simulink model "test"  (R2017a)
settings: Solver=FixedStepAuto  StartTime=0.0  StopTime=Inf  FixedStep=5e-4  RelTol=1e-3  EnableMultiTasking=on
libraries: simulink x1
settings Model: SimulationMode=external  ExtModeTrigDuration=1000000  Creator=bbb  LastModifiedBy=Nils
settings DataIOCC: LimitDataPoints=on  SaveFormat=Array
settings OptimizationCC: PassReuseOutputArgsAs=Individual arguments
settings DebuggingCC: SolverPrmCheckMsg=warning  ParameterTunabilityLossMsg=error  SFUnexpectedBacktrackingDiag=warning  SFNoUnconditionalDefaultTransitionDiag=warning  SFExecutionAtInitializationDiag=none
settings HardwareCC: ProdBitPerPointer=32  ProdBitPerSizeT=32  ProdBitPerPtrDiffT=32  ProdLargestAtomicFloat=None  ProdIntDivRoundTo=Undefined  ProdEndianess=Unspecified  ProdWordSize=32  ProdHWDeviceType=32-bit Generic
settings ModelReferenceCC: PropagateSignalLabelsOutOfModel=off
settings SFSimCC: MATLABDynamicMemAlloc=off
settings RTWCC: SystemTargetFile=ert.tlc  TemplateMakefile=ert_default_tmf  Description=Embedded Coder  RetainRTWFile=on  Toolchain=MinGW64 v4.x | gmake (64-bit Windows)  BuildConfiguration=Specify  TargetLang=C++
settings CodeAppCC: ForceParamTrailComments=on  IgnoreCustomStorageClasses=off  OperatorAnnotations=on  SimulinkDataObjDesc=on  SFDataObjDesc=on  MATLABFcnDesc=on  InsertBlockDesc=on  MATLABSourceComments=on
settings ERTTargetCC: GenerateSampleERTMain=on  SupportContinuousTime=on  ExtMode=on  ERTCustomFileTemplate=windows_file_process.tlc
settings ConfigComp: CovMetricSettings=dw  CovHtmlReporting=on  CovSaveCumulativeToWorkspaceVar=on  CovSaveSingleToWorkspaceVar=on  CovExternalEMLEnable=off  CovSFcnEnable=off

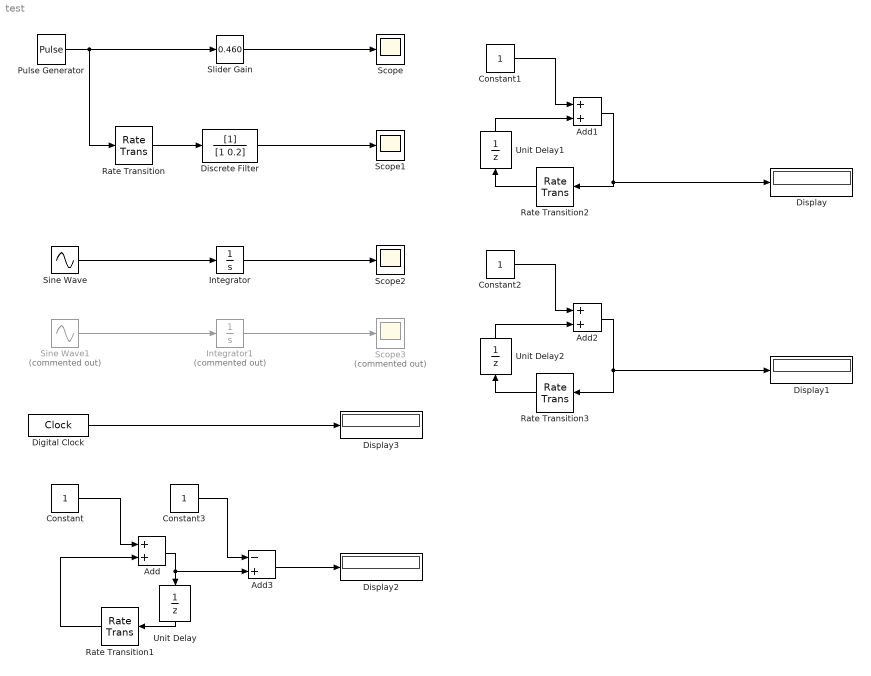
== system test ==
  Add : Sum
  Add1 : Sum
  Add2 : Sum
  Add3 : Sum  Inputs=-+
  Constant{,1..3} (4 alike) : Constant
  Digital Clock : DigitalClock
  Discrete Filter : DiscreteFilter  Denominator=[1 0.2]
  Display{,1..3} (4 alike) : Display
  Integrator : Integrator
  Integrator1 : Integrator  Commented=on
  Pulse Generator : DiscretePulseGenerator  PulseType=Time based  Amplitude=2  Period=1  PulseWidth=5
  Rate Transition : RateTransition  OutPortSampleTime=0.001
  Rate Transition1 : RateTransition  OutPortSampleTime=1
  Rate Transition2 : RateTransition  OutPortSampleTime=0.01
  Rate Transition3 : RateTransition  OutPortSampleTime=0.1
  Scope : Scope
  Scope1 : Scope
  Scope2 : Scope
  Scope3 : Scope  Commented=on
  Sine Wave : Sin  SampleTime=0
  Sine Wave1 : Sin  Commented=on  SampleTime=0.02
  Slider Gain : simulink/Math Operations/Slider Gain  gain=0.460  low=0  high=2
  Unit Delay : UnitDelay  SampleTime=-1
  Unit Delay1 : UnitDelay  SampleTime=-1
  Unit Delay2 : UnitDelay  SampleTime=-1
  wires:
  Pulse Generator/1 -> Rate Transition/1, Slider Gain/1
  Rate Transition/1 -> Discrete Filter/1
  Discrete Filter/1 -> Scope1/1
  Slider Gain/1 -> Scope/1
  Sine Wave/1 -> Integrator/1
  Integrator/1 -> Scope2/1
  Integrator1/1 -> Scope3/1
  Sine Wave1/1 -> Integrator1/1
  Constant/1 -> Add/1
  Rate Transition1/1 -> Add/2
  Add1/1 -> Display/1, Rate Transition2/1
  Constant1/1 -> Add1/1
  Unit Delay1/1 -> Add1/2
  Rate Transition2/1 -> Unit Delay1/1
  Add2/1 -> Display1/1, Rate Transition3/1
  Rate Transition3/1 -> Unit Delay2/1
  Constant2/1 -> Add2/1
  Unit Delay2/1 -> Add2/2
  Add/1 -> Add3/2, Unit Delay/1
  Digital Clock/1 -> Display3/1
  Unit Delay/1 -> Rate Transition1/1
  Constant3/1 -> Add3/1
  Add3/1 -> Display2/1
